simulink model "untitled"  (R2021a)
settings: Solver=VariableStepAuto  StartTime=0.0  StopTime=10.0  RelTol=1e-3
settings Model: OrderedModelArguments=off  Creator=duart  LastModifiedBy=duart

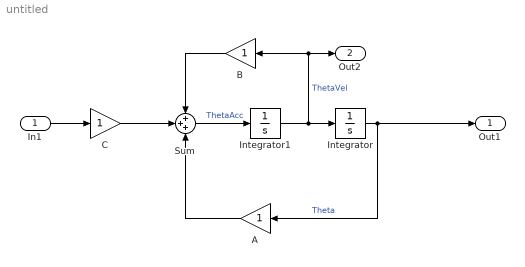
== system untitled ==
  In1 : Inport
  A : Gain
  B : Gain  ParamMin=-1000  ParamMax=1000
  C : Gain
  Integrator : Integrator
  Integrator1 : Integrator
  Sum : Sum  Inputs=+++
  Out1 : Outport
  Out2 : Outport  Port=2
  wires:
  Integrator/1 -> Out1/1, A/1  "Theta"
  Integrator1/1 -> Out2/1, B/1, Integrator/1  "ThetaVel"
  Sum/1 -> Integrator1/1  "ThetaAcc"
  A/1 -> Sum/3
  B/1 -> Sum/1
  In1/1 -> C/1
  C/1 -> Sum/2
